simulink model "Inverted_PendulumPID0"  (R2021b)
settings: Solver=ode23tb  StartTime=0.0  StopTime=30  FixedStep=0.1  RelTol=1e-3  EnableMultiTasking=on
libraries: slpidlib x1, simulink_extras x1
settings Model: Creator=Administrator  LastModifiedBy=LEE
settings SolverCC: AlgebraicLoopSolver=TrustRegion
settings DataIOCC: LimitDataPoints=on  ReturnWorkspaceOutputs=off
settings OptimizationCC: LifeSpan=inf
settings DebuggingCC: AllowSymbolicDim=off  SFUnexpectedBacktrackingDiag=warning  SFNoUnconditionalDefaultTransitionDiag=warning  SFExecutionAtInitializationDiag=none  SFMachineParentedDataDiag=warning  ArithmeticOperatorsInVariantConditions=warning
settings ModelReferenceCC: PropagateSignalLabelsOutOfModel=off
settings SFSimCC: SimUseLocalCustomCode=off  CustomCodeUndefinedFunction=UseInterfaceOnly
settings RTWCC: RTWUseLocalCustomCode=off
settings CodeAppCC: StateflowObjectComments=on
settings GRTTargetCC: TargetLangStandard=C89/C90 (ANSI)
settings ConfigComp: CovMetricSettings=dw  CovSaveCumulativeToWorkspaceVar=on  CovSaveSingleToWorkspaceVar=on  CovExternalEMLEnable=off

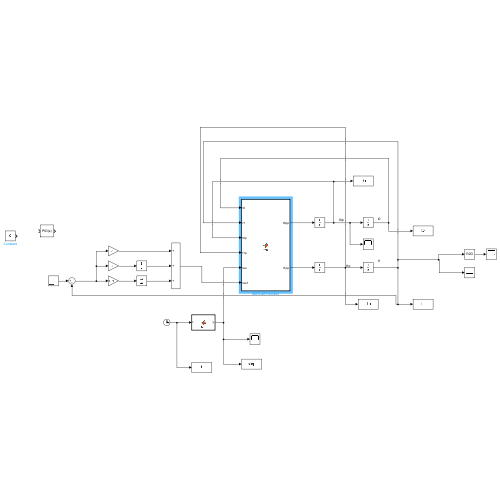
[thumbnail: Simulink's stored preview of the top-level diagram]
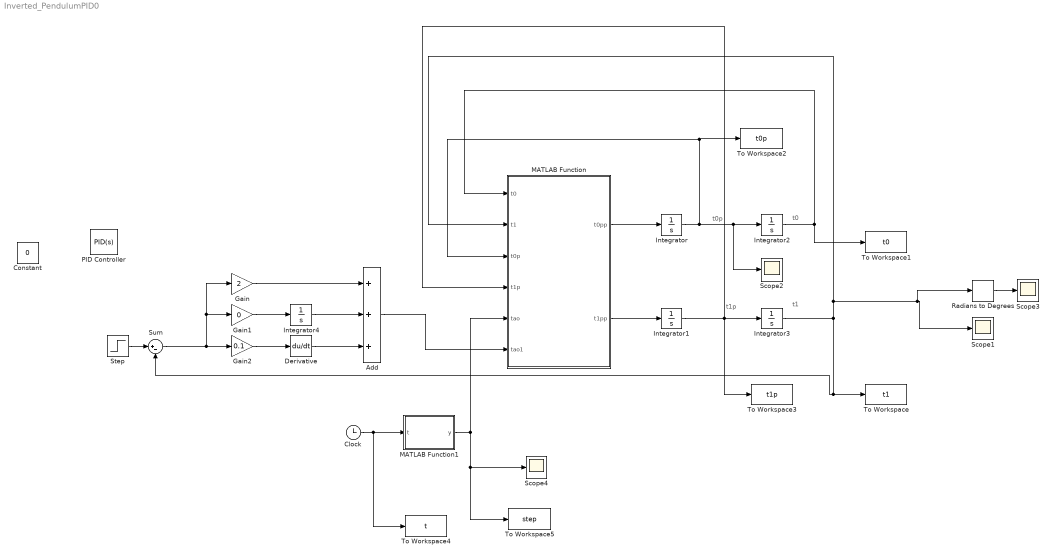
== system Inverted_PendulumPID0 ==
  note: t1
  note: t0
  note: t1p
  note: t0p
  Add : Sum  Inputs=+++
  Clock : Clock
  Constant : Constant  Value=0
  Derivative : Derivative
  Gain : Gain  Gain=2
  Gain1 : Gain  Gain=0
  Gain2 : Gain  Gain=0.1
  Integrator{,1..2,4} (4 alike) : Integrator
  Integrator3 : Integrator  InitialCondition=pi
  MATLAB Function : MATLAB Function  TreatAsAtomicUnit=on
  MATLAB Function1 : MATLAB Function  TreatAsAtomicUnit=on
  PID Controller : slpidlib/PID Controller  Controller=PID  Form=Parallel  TimeDomain=Continuous-time  UseExternalTs=off  SampleTime=-1  IntegratorMethod=Forward Euler  FilterMethod=Forward Euler  ControllerParametersSource=internal  P=2  I=0  D=1  UseFilter=on  N=100  TunerSelectOption=Transfer Function Based (PID Tuner App)  InitialConditionSource=internal  InitialConditionForIntegrator=0  InitialConditionForFilter=0  DifferentiatorICPrevScaledInput=0  ExternalReset=none  TrackingMode=off  Kt=1  LimitOutput=off  SatLimitsSource=internal  UpperSaturationLimit=inf  LowerSaturationLimit=-inf  LinearizeAsGain=on  AntiWindupMode=none  Kb=1  POutMin=[]  POutMax=[]  IOutMin=[]  IOutMax=[]  DOutMin=[]  DOutMax=[]  NOutMin=[]  NOutMax=[]  SumOutMin=[]  SumOutMax=[]  SaturationOutMin=[]  SaturationOutMax=[]  PParamMin=[]  PParamMax=[]  IParamMin=[]  IParamMax=[]  DParamMin=[]  DParamMax=[]  NParamMin=[]  NParamMax=[]  KbParamMin=[]  KbParamMax=[]  KtParamMin=[]  KtParamMax=[]  KbOutMin=[]  KbOutMax=[]  KtOutMin=[]  KtOutMax=[]  IntegratorOutMin=[]  IntegratorOutMax=[]  FilterOutMin=[]  FilterOutMax=[]  SumI1OutMin=[]  SumI1OutMax=[]  SumI2OutMin=[]  SumI2OutMax=[]  SumI3OutMin=[]  SumI3OutMax=[]  SumI4OutMin=[]  SumI4OutMax=[]  SumDOutMin=[]  SumDOutMax=[]  DifferentiatorOutMin=[]  DifferentiatorOutMax=[]  FilterDiffOutCoefMin=[]  FilterDiffOutCoefMax=[]  ReciprocalOutMin=[]  ReciprocalOutMax=[]  SumDenOutMin=[]  SumDenOutMax=[]  SumNumOutMin=[]  SumNumOutMax=[]  DivideOutMin=[]  DivideOutMax=[]  UdiffTsProdOutMin=[]  UdiffTsProdOutMax=[]  NTsProdOutMin=[]  NTsProdOutMax=[]  UintegralTsProdOutMin=[]  UintegralTsProdOutMax=[]  UngainTsProdOutMin=[]  UngainTsProdOutMax=[]  IntegratorContinuousStateAttributes=''  IntegratorStateMustResolveToSignalObject=off  IntegratorRTWStateStorageClass=Auto  FilterContinuousStateAttributes=''  FilterStateMustResolveToSignalObject=off  FilterRTWStateStorageClass=Auto  ParallelPVariant=InternalParameters  IdealPVariant=Disabled  IVariant=InternalParameters  DVariant=InternalParameters  IntegratorVariant=Continuous  SatVariant=Disabled  AWVariant=Passthrough  PCopyVariant=Disabled  TRVariant=Disabled  FdbkBlocksVariant=Forward  IdealPFdbkVariant=Disabled  SatFdbkVariant=Disabled  DerivativeFilterVariant=ContFilter  NVariant=InternalParameters  NCopyVariant=Disabled  FilterICVariant=InternalICsFilter  IntegratorICVariant=InternalICs  ExternalResetVariant=Disabled  TRSumVariant=Passthrough  SumFdbkVariant=Disabled  SumVariant=Sum_PID  TsampFilterVariant=InternalTs  TsampNgainVariant=Passthrough  TsampIntegralVariant=Passthrough  ExternalSaturationOutDataTypeStr=Inherit: Same as second input
  Radians to Degrees : simulink_extras/Transformations/Radians to Degrees
  Scope{1..4} (4 alike) : Scope
  Step : Step  After=0  SampleTime=0
  Sum : Sum  Inputs=|+-
  To Workspace : ToWorkspace  VariableName=t1  SampleTime=-1
  To Workspace1 : ToWorkspace  VariableName=t0  SampleTime=-1
  To Workspace2 : ToWorkspace  VariableName=t0p  SampleTime=-1
  To Workspace3 : ToWorkspace  VariableName=t1p  SampleTime=-1
  To Workspace4 : ToWorkspace  VariableName=t  SampleTime=-1
  To Workspace5 : ToWorkspace  VariableName=step  SampleTime=-1
  wires:
  MATLAB Function/1(t0pp) -> Integrator/1
  MATLAB Function/2(t1pp) -> Integrator1/1
  Integrator/1 -> To Workspace2/1, MATLAB Function/3(t0p), Scope2/1, Integrator2/1
  Integrator1/1 -> To Workspace3/1, Integrator3/1, MATLAB Function/4(t1p)
  Integrator2/1 -> To Workspace1/1, MATLAB Function/1(t0)
  Integrator3/1 -> Radians to Degrees/1, Scope1/1, MATLAB Function/2(t1), Sum/2, To Workspace/1
  Clock/1 -> To Workspace4/1, MATLAB Function1/1(t)
  MATLAB Function1/1(y) -> MATLAB Function/5(tao), To Workspace5/1, Scope4/1
  Add/1 -> MATLAB Function/6(tao1)
  Sum/1 -> Gain/1, Gain1/1, Gain2/1
  Gain/1 -> Add/1
  Gain1/1 -> Integrator4/1
  Integrator4/1 -> Add/2
  Gain2/1 -> Derivative/1
  Derivative/1 -> Add/3
  Step/1 -> Sum/1
  Radians to Degrees/1 -> Scope3/1

== matlab function Inverted_PendulumPID0/MATLAB Function1 ==
  data: t input; y output
function y = fcn(t)
%#codegen
if t<0.2
    y=0.5;
else
    y=0;
end

== matlab function Inverted_PendulumPID0/MATLAB Function ==
  data: t0 input; t0pp output; t1 input; t0p input; t1p input; tao input; t1pp output; tao1 input
function [t0pp,t1pp] = fcn(t0,t1,t0p,t1p,tao,tao1)
%parameters
I0=0.0052;I1=0.0023;
m1=0.2866;g=9.8;
L0=0.201;l1=0.30997;
A11=I0+m1*(L0^2)+(l1^2)*m1*(sin(t1)^2);
A12=L0*l1*m1*cos(t1);
A21=L0*l1*m1*cos(t1);
A22=I1+m1*(l1^2);
B11=2*(l1^2)*m1*sin(t1)*cos(t1)*t1p;
B12=-L0*l1*m1*sin(t1)*t1p;
B21=-(l1^2)*m1*sin(t1)*cos(t1)*t0p;
B22=0.01;
D11=0;D21=-g*l1*m1*sin(t1);
a=A11;b=A12;c=-B11*t0p-B12*t1p+tao+tao1;%
d=A21;e=A22;f=-B21*t0p-B22*t1p-D21;
t1pp=(c*d-a*f)/(b*d-a*e);
%t0pp=(c*e-b*f)/(a*e-b*d);
t0pp=(c-b*t1pp)/a;
